simulink model "ADAS_Main"  (R2026a)
settings: Solver=FixedStepDiscrete  StopTime=5
InitFcn:
  | createLidarActorProfiles;
model workspace (MAT data in the model file):
  firstWarning = 1
  originalScenarioChecksum = '71EAF3DF157DF5A35F75811B676F8B0F'
undefined symbols (not defined in the file): driving, matlabshared
libraries: drivingscenarioandsensors x3, lidarlib x1
(part 4 of 6)

== matlab function ADAS_Main/Tracking_Prediction/Track_Lifecycle ==
  data: iState input; oState output; iCov input; iID input; iStatus input; iNextID input; iHits input; iTsu input; iR1 input; prevWin input uint32 size=512 1; prevAge input uint32 size=512 1; prevLost input double size=512 10; oCov output; oID output; oStatus output; oNextID output; oHits output; oTsu output; oR1 output; oWin output; oAge output; oLost output; lifeDiag output; iAttr input double size=512 3; oAttr output; oTrackAttributes output
function [oState, oCov, oID, oStatus, oNextID, oHits, oTsu, oR1, ...
          oWin, oAge, oLost, lifeDiag, oAttr, oTrackAttributes] = ...
    Track_Lifecycle(iState, iCov, iID, iStatus, iNextID, iHits, iTsu, iR1, ...
                    prevWin, prevAge, prevLost, iAttr)
%#codegen
% TRACK_LIFECYCLE  Stage 5: track lifecycle ONLY.
%   FREE -> TENTATIVE -> CONFIRMED -> COASTED -> LOST -> deleted (slot to FREE)
%
% THIS BLOCK DOES NOT: observe velocity, estimate acceleration, keep history,
% emit prediction horizons, rank threats, or make any manoeuvre decision.
% It does not touch the state estimate: it only changes STATUS and bookkeeping,
% and moves records between the active and lost tables.
%
% VELOCITY OBSERVATION REMAINS UNTOUCHED AND UNDECIDED. Velocity is never
% zeroed, never re-estimated and never used as a lifecycle criterion here.
%
% PLACEMENT: runs AFTER Track_Update, so Track_Update stays byte-identical
% (Stage-4 corrections are frozen). Its output feeds the Unit Delays.
%
% "MATCHED THIS FRAME" is detected as iTsu == 0. Track_Update sets tsu to 0 on a
% successful update and to prevTsu+dt otherwise, and a newly born track also has
% tsu 0 - which is correct, since birth is its first hit.
%
% CONFIRMATION - 2 of 3, NOT 2 consecutive
%   oWin is a 3-bit shift register, bit0 = most recent frame, 1 = hit.
%       win = bitand(bitshift(prevWin,1) + matched, 7)
%   CONFIRM  when popcount(win) >= 2
%   DELETE   when (age >= 2 and the last two frames are both misses)
%            or  (age >= 3 and popcount(win) < 2)   <- window closed, <2 hits
%   Confirmation is tested BEFORE deletion. Verified against all six frozen
%   sequences: hit-hit, hit-miss-hit, miss-hit-hit confirm; hit-miss-miss,
%   miss-hit-miss, miss-miss-* delete.
%
% COASTING
%   CONFIRMED + miss -> COASTED. A coasted track keeps its predicted state,
%   its velocity, and its covariance exactly as Track Prediction left them;
%   nothing is zeroed or reset. It keeps competing for association and stays
%   reported. COASTED + match -> CONFIRMED with the SAME TrackID.
%
% COASTED -> LOST (frozen criterion, no threat input)
%   sigma_assoc = sqrt(max(P11,P22)) of the current (predicted) covariance.
%   LOST when  KGATE * sigma_assoc >= WLANE  (3.03 * sigma >= 3.5 m).
%   The record is MOVED to the lost table and the active slot returns to FREE,
%   so a LOST record cannot participate in association - Track_Association
%   iterates the active table only and therefore needed no change.
%
% LOST retention (frozen, literal)
%   delete when TimeSinceUpdate >= T_LOST = 1.5 s.
%   NOTE: TimeSinceUpdate accumulates from the track's LAST UPDATE, not from
%   the moment it became LOST, so this gives 1.5 s of total post-update
%   retention rather than 1.5 s in addition to the coasting phase. This is the
%   literal frozen rule; the measured consequence is reported at the checkpoint.
%
% REACQUISITION - two different things
%   1. COASTED gets a match  -> CONFIRMED, SAME TrackID. Counted in NumReacquired.
%   2. A LOST object physically reappears -> must become a NEW track with a NEW
%      TrackID. NOT IMPLEMENTABLE HERE: recognising that a detection corresponds
%      to a lost record requires comparing it against the lost table, which is
%      association with LOST records and is explicitly forbidden. No flag is
%      fabricated. Reported as an open item.
%
% TrackID is uint32, monotonic, never reused, independent of slot index. A
% deleted or lost record never returns its ID to circulation.
%
% NO EVICTION anywhere: neither the active table nor the lost table ever removes
% an existing record to make room. Overflow is reported instead.
%
% SCENARIO INDEPENDENCE: consumes only track state, covariance and timing. No
% actor identity, class, count, trajectory, map or scenario geometry.

MAX_T  = 512;
MAX_L  = 512;          % MAX_TRACKS_LOST
NCOL_L = 10;
DT     = 0.1;
KGATE  = 3.03;
WLANE  = 3.5;
T_LOST = 1.5;
V_CONV = 0.875;

ST_FREE = uint8(0); ST_TENT = uint8(1); ST_CONF = uint8(2); ST_COAST = uint8(3);

oState  = zeros(MAX_T,4);
oCov    = zeros(MAX_T,10);
oID     = zeros(MAX_T,1,'uint32');
oStatus = zeros(MAX_T,1,'uint8');
oHits   = zeros(MAX_T,1,'uint32');
oTsu    = zeros(MAX_T,1);
oR1     = zeros(MAX_T,3);
% ---- additive: persistent LiDAR extent attributes, and the ICE-facing output --
% oAttr           [512x3]  state fed back through the Unit Delay
% oTrackAttributes[512x4]  Valid | Length | Width | TrustFlags
% A freed slot falls through the ~keep continue below, so BOTH arrays stay
% exactly zero for it. No extent is invented and no default size substituted.
oAttr            = zeros(MAX_T,3);
oTrackAttributes = zeros(MAX_T,4);
oWin    = zeros(MAX_T,1,'uint32');
oAge    = zeros(MAX_T,1,'uint32');
oLost   = zeros(MAX_L,NCOL_L);
oNextID = iNextID;
lifeDiag = zeros(1,12);

% ---- 1. age the lost table and retire expired records --------------------
nLostDel = 0;
for k = 1:MAX_L
    if prevLost(k,1) == 0
        continue                            % free lost slot
    end
    tsuL = prevLost(k,9) + DT;
    if tsuL >= T_LOST
        nLostDel = nLostDel + 1;            % retired; TrackID never returns
        continue
    end
    for c = 1:NCOL_L
        oLost(k,c) = prevLost(k,c);
    end
    oLost(k,9) = tsuL;
end

% ---- 2. lifecycle transitions on the active table ------------------------
nTent = 0; nConf = 0; nCoast = 0; nDelT = 0; nConfTr = 0; nReacq = 0;
nToLost = 0; lostOvf = 0; nLostDrop = 0; nConv = 0; nExpOnEntry = 0;

for t = 1:MAX_T
    st = iStatus(t);
    if st == ST_FREE
        continue                            % slot stays entirely zero
    end

    matched = 0;
    if iTsu(t) == 0
        matched = 1;
    end
    w  = bitand(bitshift(uint32(prevWin(t)),1) + uint32(matched), uint32(7));
    ag = prevAge(t) + uint32(1);
    pc = bitand(w,uint32(1)) + bitand(bitshift(w,-1),uint32(1)) + bitand(bitshift(w,-2),uint32(1));

    keep = true;
    toLost = false;

    if st == ST_TENT
        if pc >= 2
            st = ST_CONF; nConfTr = nConfTr + 1;
        elseif (ag >= 2 && bitand(w,uint32(3)) == 0) || (ag >= 3 && pc < 2)
            keep = false; nDelT = nDelT + 1;
        end
    elseif st == ST_CONF
        if matched == 0
            st = ST_COAST;
        end
    else                                    % ST_COAST
        if matched == 1
            st = ST_CONF; nReacq = nReacq + 1;
        end
    end

    if keep && st == ST_COAST
        s1 = iCov(t,1); s2 = iCov(t,5);
        sm = s1; if s2 > sm, sm = s2; end
        if sm < 0, sm = 0; end
        if KGATE*sqrt(sm) >= WLANE
            toLost = true; keep = false;
        end
    end

    if toLost && iTsu(t) >= T_LOST
        % already past the retention limit at the moment of transfer - the
        % literal rule retires it immediately rather than holding it a frame
        nLostDel = nLostDel + 1;
        nExpOnEntry = nExpOnEntry + 1;
        toLost = false;
    end

    if toLost
        slot = 0;
        for k = 1:MAX_L
            if oLost(k,1) == 0, slot = k; break; end
        end
        if slot == 0
            lostOvf = 1; nLostDrop = nLostDrop + 1;   % NEVER evict an existing record
        else
            oLost(slot,1)  = double(iID(t));
            oLost(slot,2)  = iState(t,1);
            oLost(slot,3)  = iState(t,2);
            oLost(slot,4)  = iState(t,3);
            oLost(slot,5)  = iState(t,4);
            oLost(slot,6)  = iCov(t,1);
            oLost(slot,7)  = iCov(t,5);
            oLost(slot,8)  = iCov(t,2);
            oLost(slot,9)  = iTsu(t);
            oLost(slot,10) = double(ag);
            nToLost = nToLost + 1;
        end
    end

    if ~keep
        continue                            % slot returns to FREE (all zeros)
    end

    for c = 1:4,  oState(t,c) = iState(t,c); end
    for c = 1:10, oCov(t,c)   = iCov(t,c);   end
    for c = 1:3,  oR1(t,c)    = iR1(t,c);    end
    for c = 1:3,  oAttr(t,c)  = iAttr(t,c);  end
    oTrackAttributes(t,1) = 1;                  % Valid == post-lifecycle validity
    oTrackAttributes(t,2) = iAttr(t,1);         % Length
    oTrackAttributes(t,3) = iAttr(t,2);         % Width
    oTrackAttributes(t,4) = iAttr(t,3);         % TrustFlags, carried verbatim
    oID(t)     = iID(t);
    oStatus(t) = st;
    oHits(t)   = iHits(t);
    oTsu(t)    = iTsu(t);
    oWin(t)    = w;
    oAge(t)    = ag;

    if st == ST_TENT,  nTent  = nTent  + 1; end
    if st == ST_CONF,  nConf  = nConf  + 1; end
    if st == ST_COAST, nCoast = nCoast + 1; end
    if sqrt(iCov(t,8)) < V_CONV && sqrt(iCov(t,10)) < V_CONV
        nConv = nConv + 1;                  % derived, never a lifecycle criterion
    end
end

nLostNow = 0;
for k = 1:MAX_L
    if oLost(k,1) ~= 0, nLostNow = nLostNow + 1; end
end

lifeDiag(1)  = nTent;
lifeDiag(2)  = nConf;
lifeDiag(3)  = nCoast;
lifeDiag(4)  = nLostNow;
lifeDiag(5)  = nDelT + nLostDel;
lifeDiag(6)  = nDelT;
lifeDiag(7)  = nConfTr;
lifeDiag(8)  = nReacq;
lifeDiag(9)  = nToLost;
lifeDiag(10) = lostOvf;
lifeDiag(11) = nLostDrop;
lifeDiag(12) = nConv;

end

== matlab function ADAS_Main/Tracking_Prediction/Track_History ==
  data: trkState input; hist output; trkID input; trkStatus input; trkTsu input; simTime input; prevHist input double size=512 30 4; prevRing input uint32 size=512 1; ringIdx output; validCount output; histSpan output
function [hist, ringIdx, validCount, histSpan] = ...
    Track_History(trkState, trkID, trkStatus, trkTsu, simTime, prevHist, prevRing)
%#codegen
% TRACK_HISTORY  Stage 6: per-track temporal history ONLY.
%
% THIS BLOCK DOES NOT: estimate acceleration, emit prediction horizons, run
% Behavior/Intention, Risk, Planning or Controller, observe velocity, or do any
% LOST-track re-identification. It does not touch the state estimate, the
% lifecycle, or any Stage-3/4/5 contract - it only records where each active
% track has been.
%
% Tracking's own recursive estimator needs no history. This buffer exists to
% give Behavior/Intention temporal information downstream.
%
% LAYOUT (frozen)
%   hist [512 x 30 x 4] double   channel 1 = X
%                                channel 2 = Y
%                                channel 3 = Valid (1 measured, 0 predicted)
%                                channel 4 = timestamp (s, actual sim time)
%   30 samples at dt = 0.1 s  ->  3.0 s of coverage.
%   ringIdx [512 x 1] uint32     index of the MOST RECENT sample, 1..30; 0 = empty
%
% RING BEHAVIOUR
%   The ring advances EVERY frame for every active track, whether or not a
%   measurement arrived. The temporal grid therefore stays uniform:
%   t, t-dt, t-2dt, ... Valid samples are never compacted together, so a gap
%   remains visible as a run of Valid = 0 rather than being closed up.
%   On the 31st write the oldest sample is overwritten deterministically.
%
% VALID
%   Valid = 1 only when the track received a measurement this frame, detected as
%   trkTsu == 0 (Track_Update zeroes it on a successful update and on birth).
%   A COASTED track - or a TENTATIVE track that missed - still gets a sample
%   written with its PREDICTED X/Y, but marked Valid = 0. A prediction is never
%   recorded as a measurement.
%
% STATUS INDEPENDENCE
%   Storage does not depend on confirmation status. TENTATIVE, CONFIRMED and
%   COASTED tracks all keep history. History is never deleted for being
%   unconfirmed, and never ranked or filtered - every active slot has its own
%   independent buffer.
%
% FREE SLOTS AND SLOT REUSE
%   A slot whose status is FREE has its entire history zeroed and ringIdx set to
%   0. Because Track_Lifecycle frees a slot in the very output this block
%   consumes, the FREE state is always observed before any new track can occupy
%   that slot, so a new occupant always starts from a cleared buffer. Old and
%   new trajectories are therefore never spliced.
%
% LOST
%   A track entering LOST leaves the active table, so its slot reads FREE here
%   and its history is discarded. No history is kept for LOST records and none
%   is ever carried into a future track.
%
% TrackID vs SLOT
%   History follows the SLOT. trkID is carried only so downstream can label the
%   buffer; it is never assumed equal to the slot index.
%
% DERIVED METADATA (the only two exposed at this stage)
%   validCount [512 x 1]  number of Valid == 1 samples, 0..30. Coasted and
%                         empty samples are NOT counted.
%   histSpan   [512 x 1]  newest valid timestamp minus oldest valid timestamp,
%                         computed from the STORED TIMESTAMPS, not from the
%                         valid-sample count. Fewer than two valid samples -> 0.
%                         So valid,valid,invalid,invalid,valid spans 0.4 s, not
%                         the 0.2 s a count-based formula would give.
%
% SCENARIO INDEPENDENCE: consumes only track state, status, timing and the
% simulation clock. No actor identity, class, count, map or scenario geometry.

MAX_T = 512;
NS    = 30;

hist       = zeros(MAX_T, NS, 4);
ringIdx    = zeros(MAX_T, 1, 'uint32');
validCount = zeros(MAX_T, 1);
histSpan   = zeros(MAX_T, 1);

ts = simTime;
if ~isfinite(ts), ts = 0; end

for t = 1:MAX_T
    if trkStatus(t) == 0
        continue                    % FREE: history and ring stay exactly zero
    end

    % ---- advance the ring every frame, measured or not
    ri = double(prevRing(t)) + 1;
    if ri > NS, ri = 1; end
    if ri < 1,  ri = 1; end

    for s = 1:NS
        for c = 1:4
            hist(t,s,c) = prevHist(t,s,c);
        end
    end

    vflag = 0;
    if trkTsu(t) == 0
        vflag = 1;                  % measured this frame
    end
    hist(t,ri,1) = trkState(t,1);
    hist(t,ri,2) = trkState(t,2);
    hist(t,ri,3) = vflag;
    hist(t,ri,4) = ts;
    ringIdx(t)   = uint32(ri);

    % ---- derived metadata, from the stored timestamps
    nv = 0; tmin = 0; tmax = 0; first = true;
    for s = 1:NS
        if hist(t,s,3) == 1
            nv = nv + 1;
            tv = hist(t,s,4);
            if first
                tmin = tv; tmax = tv; first = false;
            else
                if tv < tmin, tmin = tv; end
                if tv > tmax, tmax = tv; end
            end
        end
    end
    validCount(t) = nv;
    if nv >= 2
        histSpan(t) = tmax - tmin;
    else
        histSpan(t) = 0;
    end
end

end

== matlab function ADAS_Main/Tracking_Prediction/Prediction_Horizons ==
  data: trkState input; trkPred output; trkCov input; trkStatus input
function trkPred = Prediction_Horizons(trkState, trkCov, trkStatus)
%#codegen
% PREDICTION_HORIZONS  Stage 7: pure kinematic projection of each active track
% onto a fixed ladder of future times. NOTHING ELSE.
%
% THIS BLOCK DOES NOT: estimate acceleration, fit anything to Track History,
% classify manoeuvres, produce lane-change / braking / cut-in / overtaking
% likelihoods, compute TTC, collision probability, risk or threat, or propose
% ego trajectories. Those belong to Behavior/Intention, the Risk Engine and
% Planning respectively. It answers only "where could this object be under the
% existing CV model", never "what will it choose to do".
%
% It is a PURE FUNCTION of the current track state - stateless, no Unit Delay.
% It does not modify Track_History, Track_Lifecycle, Track_Update or any
% Stage-3..6 contract, and velocity observation is untouched.
%
% EGO FRAME
%   The input state is already expressed in the current ego-compensated frame.
%   No further ego compensation is applied, no future ego motion is assumed, and
%   no ego manoeuvre is presumed. Outputs are target states relative to the
%   CURRENT compensated tracking frame.
%
% MEAN
%   x_h = F(h)*x ,  F(h) = [1 0 h 0; 0 1 0 h; 0 0 1 0; 0 0 0 1]
%
% COVARIANCE - OPTION B (approved): exact closed-form evaluation of the
% ALREADY FROZEN discrete-time model. This is NOT a new covariance model; it is
% the algebraic value of
%       P_N = F^N P (F^N)' + sum_{j=0}^{N-1} F^j Q(dt) (F^j)'
% computed without numerically iterating. With a = dt^4/4, b = dt^3/2, c = dt^2
% and N = h/dt (exactly integral for all seven horizons: 5 10 15 20 30 40 50):
%       Q11 = q*[ N*a + b*dt*N*(N-1) + c*dt^2*(N-1)*N*(2*N-1)/6 ]
%       Q12 = q*[ N*b + c*dt*N*(N-1)/2 ]
%       Q22 = q*[ N*c ]
%   Verified against explicit repeated Q(dt) propagation on all 16 elements and
%   all seven horizons: max |dQ| 2.13e-14, max |dP| 7.11e-15, and over 500
%   random PD covariances max |dP| 4.55e-13.
%
%   The single-step form q*h^4/4 is DELIBERATELY NOT USED - it does not match the
%   frozen Stage-2 discrete process model and would inflate sigma at 5 s from
%   6.48 m to 37.56 m.
%
% OUTPUT  trkPred [512 x 7 x 7] double, indexed (track, horizon, field)
%   horizon index 1..7 -> 0.5 1.0 1.5 2.0 3.0 4.0 5.0 s
%   field   index 1..7 -> 1 X, 2 Y, 3 Vx, 4 Vy, 5 PosCovXX, 6 PosCovYY, 7 PosCovXY
%   Both trailing dimensions are 7; the ordering above is the contract.
%
% COVERAGE
%   Every ACTIVE track is predicted - TENTATIVE, CONFIRMED and COASTED alike.
%   No ranking, no filtering, no "primary target", no nearest/front/highest-score
%   selection. If 107 tracks are active, all 107 get the full ladder. LOST tracks
%   are not in the active table and so receive nothing. FREE rows stay zero.
%
% UNCERTAINTY
%   Covariance grows naturally with the horizon and is never clamped, shrunk or
%   cosmetically adjusted, and a large covariance is never a reason to drop a
%   track - lifecycle already made that call. A track with
%   VelocityConverged = false keeps its large velocity covariance, which
%   propagates into the position covariance exactly as the model dictates; its
%   Vx = Vy = 0 placeholder is NOT treated as stationary and its future velocity
%   is NOT zeroed. Downstream interprets the uncertainty.
%
% SCENARIO INDEPENDENCE: consumes only track state, covariance and status. No
% actor identity, class, count, map or scenario geometry.

MAX_T = 512;
NH    = 7;
NFLD  = 7;
DT    = 0.1;
QA    = 9.0;                 % m^2/s^4, frozen
P_FLOOR_POS = 1e-6;          % existing floor, applied only if violated

trkPred = zeros(MAX_T, NH, NFLD);

hor = [0.5 1.0 1.5 2.0 3.0 4.0 5.0];
aa = DT^4/4;  bb = DT^3/2;  cc = DT^2;

for k = 1:NH
    h = hor(k);
    N = h/DT;
    Nr = floor(N + 0.5);
    if Nr < 1, Nr = 1; end
    Nd = double(Nr);

    q11 = QA*( Nd*aa + bb*DT*Nd*(Nd-1) + cc*DT*DT*(Nd-1)*Nd*(2*Nd-1)/6 );
    q12 = QA*( Nd*bb + cc*DT*Nd*(Nd-1)/2 );   %#ok<NASGU> same-axis pos/vel term,
    % retained for documentation of the full Q_acc; the position block only
    % needs Q_acc(1,1)=q11 and Q_acc(2,2)=q11, and Q_acc(1,2)=0.
    q22 = QA*( Nd*cc );

    for t = 1:MAX_T
        if trkStatus(t) == 0
            continue                     % FREE row stays zero
        end

        x1 = trkState(t,1); x2 = trkState(t,2);
        x3 = trkState(t,3); x4 = trkState(t,4);

        p11 = trkCov(t,1); p12 = trkCov(t,2); p13 = trkCov(t,3); p14 = trkCov(t,4);
        p22 = trkCov(t,5); p23 = trkCov(t,6); p24 = trkCov(t,7);
        p33 = trkCov(t,8); p34 = trkCov(t,9); p44 = trkCov(t,10);

        % ---- mean: x_h = F(h)*x
        m1 = x1 + h*x3;
        m2 = x2 + h*x4;
        m3 = x3;
        m4 = x4;

        % ---- position block of F(h)*P*F(h)' , then + Q_acc
        c11 = p11 + 2*h*p13 + h*h*p33 + q11;
        c22 = p22 + 2*h*p24 + h*h*p44 + q11;
        % NOTE: Q_acc(1,2) is ZERO - q12 is the position/velocity cross term of
        % the SAME axis (Q_acc(1,3)), not the x-y position cross term. It must
        % NOT be added here.
        c12 = p12 + h*p14 + h*p23 + h*h*p34;

        if ~isfinite(c11) || c11 < P_FLOOR_POS, c11 = P_FLOOR_POS; end
        if ~isfinite(c22) || c22 < P_FLOOR_POS, c22 = P_FLOOR_POS; end
        if ~isfinite(c12), c12 = 0; end
        if ~isfinite(m1), m1 = 0; end
        if ~isfinite(m2), m2 = 0; end
        if ~isfinite(m3), m3 = 0; end
        if ~isfinite(m4), m4 = 0; end

        trkPred(t,k,1) = m1;
        trkPred(t,k,2) = m2;
        trkPred(t,k,3) = m3;
        trkPred(t,k,4) = m4;
        trkPred(t,k,5) = c11;
        trkPred(t,k,6) = c22;
        trkPred(t,k,7) = c12;
    end
end

end

== matlab function ADAS_Main/Behavior_ICE/ICE_Evaluate ==
  data: TrackState input; Verdict3 output; TrackCov input; TrackID input; TrackStatus input; TrackAttributes input; EgoKinematics input; M_adm output; N_adm output; N_inadm output; InadmIDs output; InadmReason output; InadmOverflow output; AdmVacuous output; Bind output; N_active output; N_clear output; M_res output; ResVacuous output
function [Verdict3, M_adm, N_adm, N_inadm, InadmIDs, InadmReason, ...
          InadmOverflow, AdmVacuous, Bind, N_active, N_clear, M_res, ResVacuous] = ...
    ICE_Evaluate(TrackState, TrackCov, TrackID, TrackStatus, TrackAttributes, EgoKinematics) %#codegen
%ICE_EVALUATE  Fixed-size ICE, Simulink MATLAB Function compatible.
%
%   Functionally equivalent to ice_adm(ice_core(...)). The reference pair
%   ice_core.m / ice_adm.m / ice_par.m remains the ORACLE; this file must
%   reproduce them. No mathematics, parameter, semantic or threshold changed.
%
%   FIXED SIZE ONLY. No find(), no unique(), no sort(), no varsize, no heap.
%   See ICE_FIXEDSIZE_NOTES in the design document for the three replacements.
%
%   Ego model, per approved decisions:
%     egoV   = EgoKinematics(1)   planar ego speed        (D3)
%     egoPsi = 0                  pinned interface invariant (D5)
%     straight nominal candidate lattice                   (D4)
%     EgoKinematics(2) (yaw rate) carried but NOT consumed (D5/approved item 5)

%% ---- constants, copied VERBATIM from ice_par.m -------------------------
NT   = 512;                                   % PAR.capN
HS   = [0.5 1.0 1.5 2.0 3.0 4.0 5.0];         % PAR.hs
H    = 7;
O    = 4;                                     % PAR.O
NANG = 8;                                     % PAR.nAng
NRAD = 4;                                     % PAR.nRad
MC   = NANG*NRAD;                             % 32 candidates per sector
CLEVEL = 9.21;
U      = 8.0;
VMAX   = 40.0;
U_EGO  = 8.0;
R_EGO  = 3.9906;
ASPECT = 10.0;
OCCL   = 2.0;
UNTRUST= 2.0;
THINFL = 0.6;
ACTTOL = 1e-9;
BC     = 8;                                   % PAR.bindCap
IC     = 32;                                  % InadmIDs capacity (approved)
NOAGENT= inf;                                 % PAR.noAgentMargin
FL_THIN      = 4;
FL_UNTRUSTED = 8;

EGOV   = EgoKinematics(1);                    % D3
% egoPsi is pinned to 0 (D5). The rotation R(-0) is the exact identity, so
% it is omitted rather than multiplied; equivalence is asserted by test.

%% ---- outputs preallocated (fixed size) ---------------------------------
Verdict3      = zeros(O,H,'int8');
M_adm         = zeros(O,H);
N_active      = zeros(O,H,'uint16');
N_clear       = zeros(O,H,'uint16');
M_res         = zeros(O,H);
ResVacuous    = false(O,H);
Bind          = zeros(O,H,BC,'uint32');
InadmIDs      = zeros(IC,1,'uint32');
InadmReason   = zeros(IC,1,'uint8');
InadmOverflow = false;

%% ---- stage 1: admissibility over ALL 512 slots -------------------------
% Reason bits: 1 EXTENT | 2 COVARIANCE | 4 OTHER
live   = false(NT,1);
reason = zeros(NT,1,'uint8');
for t = 1:NT
    if TrackStatus(t) == 0
        continue
    end
    live(t) = true;
    r = uint8(0);

    if TrackAttributes(t,1) ~= 1
        r = bitor(r, uint8(4));
    end

    L = TrackAttributes(t,2);
    W = TrackAttributes(t,3);
    if ~isfinite(L) || ~isfinite(W) || L <= 0 || W <= 0
        r = bitor(r, uint8(1));
    end

    p11 = TrackCov(t,1); p12 = TrackCov(t,2);
    q11 = TrackCov(t,3); q12 = TrackCov(t,4);
    p22 = TrackCov(t,5);
    q21 = TrackCov(t,6); q22 = TrackCov(t,7);
    v11 = TrackCov(t,8); v12 = TrackCov(t,9); v22 = TrackCov(t,10);
    finite10 = isfinite(p11) && isfinite(p12) && isfinite(q11) && isfinite(q12) && ...
               isfinite(p22) && isfinite(q21) && isfinite(q22) && ...
               isfinite(v11) && isfinite(v12) && isfinite(v22);
    if ~finite10 || ~isPD2f(p11,p12,p12,p22)
        r = bitor(r, uint8(2));
    else
        for k = 1:H
            h = HS(k);
            s11 = p11 + 2*h*q11 + h*h*v11;
            s12 = p12 + h*(q12 + q21) + h*h*v12;
            s22 = p22 + 2*h*q22 + h*h*v22;
            if ~isPD2f(s11,s12,s12,s22)
                r = bitor(r, uint8(2));
                break
            end
        end
    end
    reason(t) = r;
end

adm = live & (reason == 0);
nAdm = 0; nInadm = 0; nFill = 0;
for t = 1:NT
    if ~live(t), continue; end
    if reason(t) == 0
        nAdm = nAdm + 1;
    else
        nInadm = nInadm + 1;
        if nFill < IC                      % slot order; NO ranking
            nFill = nFill + 1;
            InadmIDs(nFill)    = TrackID(t);
            InadmReason(nFill) = reason(t);
        else
            InadmOverflow = true;
        end
    end
end
N_adm      = uint16(nAdm);
N_inadm    = uint16(nInadm);
AdmVacuous = (nAdm == 0);

%% ---- stage 2: per-agent envelopes, all 512 slots -----------------------
rFoot    = zeros(NT,1);
cAx = zeros(NT,H); cAy = zeros(NT,H); rA = zeros(NT,H);
cBx = zeros(NT,H); cBy = zeros(NT,H); rB = zeros(NT,H);
resolved = false(NT,H);

for t = 1:NT
    if ~adm(t), continue; end

    L = TrackAttributes(t,2);
    W = TrackAttributes(t,3);
    fl = uint32(max(TrackAttributes(t,4),0));
    base = 0.5*sqrt(L*L + W*W);
    if bitand(fl, uint32(FL_UNTRUSTED)) > 0
        base = base * UNTRUST;
    end
    if bitand(fl, uint32(FL_THIN)) > 0
        base = max(base, THINFL);
    end
    cap = ASPECT * 0.5 * min(L,W);
    rFoot(t) = min(base + OCCL, max(base, cap));

    p11 = TrackCov(t,1); p12 = TrackCov(t,2);
    q11 = TrackCov(t,3); q12 = TrackCov(t,4);
    p22 = TrackCov(t,5);
    q21 = TrackCov(t,6); q22 = TrackCov(t,7);
    v11 = TrackCov(t,8); v12 = TrackCov(t,9); v22 = TrackCov(t,10);

    r0 = sqrt(CLEVEL * lmax2f(p11,p12,p12,p22));
    for k = 1:H
        h = HS(k);
        s11 = p11 + 2*h*q11 + h*h*v11;
        s12 = p12 + h*(q12 + q21) + h*h*v12;
        s22 = p22 + 2*h*q22 + h*h*v22;
        rEpi = sqrt(CLEVEL * lmax2f(s11,s12,s12,s22));
        cAx(t,k) = TrackState(t,1) + h*TrackState(t,3);
        cAy(t,k) = TrackState(t,2) + h*TrackState(t,4);
        rA(t,k)  = rEpi + 0.5*U*h*h + rFoot(t);
        cBx(t,k) = TrackState(t,1);
        cBy(t,k) = TrackState(t,2);
        rB(t,k)  = r0 + VMAX*h + rFoot(t);
        resolved(t,k) = (rEpi < 0.5*min(L,W));
    end
end

%% ---- stage 3: candidates and max-min -----------------------------------
dA  = zeros(MC,NT);
dB  = zeros(MC,NT);
Dm  = zeros(MC,NT);
Dr  = zeros(MC,NT);
d1  = zeros(MC,1);
i1  = zeros(MC,1);
d2  = zeros(MC,1);
activeFlag = false(NT,1);
bidbuf = zeros(BC,1,'uint32');

for k = 1:H
    h      = HS(k);
    egoNom = EGOV*h;                        % D3/D4: straight nominal
    Rreach = 0.5*U_EGO*h*h;
    for o = 1:O
        w  = 2*pi/O;
        a0 = -pi + (o-1)*w;

        % ---- REPLACEMENT 1 for find(): mask, never gather -------------
        % every non-admissible column is +Inf so it can never attain a min
        for m = 1:MC
            ia = floor((m-1)/NRAD) + 1;     % meshgrid(ang,rad) column-major
            ir = m - (ia-1)*NRAD;
            ang = a0 + (ia - 0.5)*(w/NANG);
            rad = (ir/NRAD)*Rreach;
            cx  = egoNom + rad*cos(ang);
            cy  =          rad*sin(ang);
            for t = 1:NT
                if ~adm(t)
                    dA(m,t) = inf; dB(m,t) = inf; Dm(m,t) = inf; Dr(m,t) = inf;
                    continue
                end
                ax = cx - cAx(t,k); ay = cy - cAy(t,k);
                bx = cx - cBx(t,k); by = cy - cBy(t,k);
                da = hypot(ax,ay) - R_EGO - rA(t,k);
                db = hypot(bx,by) - R_EGO - rB(t,k);
                dA(m,t) = da; dB(m,t) = db;
                dm = da; if db > dm, dm = db; end
                Dm(m,t) = dm;
                if resolved(t,k), Dr(m,t) = dm; else, Dr(m,t) = inf; end
            end
        end

        % row minima and second minima
        Mv = -inf; nClear = 0;
        for m = 1:MC
            bv = inf; bi = 0;
            for t = 1:NT
                if Dm(m,t) < bv, bv = Dm(m,t); bi = t; end
            end
            d1(m) = bv; i1(m) = bi;
            sv = inf;
            for t = 1:NT
                if t == bi, continue; end
                if Dm(m,t) < sv, sv = Dm(m,t); end
            end
            d2(m) = sv;
            if bv > Mv, Mv = bv; end
            if bv > 0,  nClear = nClear + 1; end
        end

        % ---- REPLACEMENT 2 for unique(): set membership by flag -------
        for t = 1:NT, activeFlag(t) = false; end
        for m = 1:MC
            if d2(m) > Mv + ACTTOL && i1(m) > 0
                activeFlag(i1(m)) = true;
            end
        end

        % ---- REPLACEMENT 3 for sort(): bounded ascending insertion ----
        % keeps the BC smallest TrackIDs in ascending order, exactly as
        % sort(...) followed by truncation to BC does in the reference
        nb = 0; nActive = 0;
        for b = 1:BC, bidbuf(b) = uint32(0); end
        for t = 1:NT
            if ~activeFlag(t), continue; end
            nActive = nActive + 1;
            v = TrackID(t);
            pos = nb + 1;
            for b = 1:BC
                if b <= nb && v < bidbuf(b)
                    pos = b; break
                end
            end
            if pos <= BC
                last = nb; if last > BC-1, last = BC-1; end
                for b = last:-1:pos
                    bidbuf(b+1) = bidbuf(b);
                end
                bidbuf(pos) = v;
                if nb < BC, nb = nb + 1; end
            end
        end

        % resolved-agent bracket
        Mr = -inf; anyRes = false;
        for m = 1:MC
            rv = inf;
            for t = 1:NT
                if Dr(m,t) < rv, rv = Dr(m,t); end
            end
            if rv > Mr, Mr = rv; end
        end
        for t = 1:NT
            if adm(t) && resolved(t,k), anyRes = true; break; end
        end

        % ---- outputs -------------------------------------------------
        if nAdm == 0
            M_adm(o,k)      = NOAGENT;
            N_clear(o,k)    = uint16(MC);
            N_active(o,k)   = uint16(0);
        else
            M_adm(o,k)      = Mv;
            N_clear(o,k)    = uint16(nClear);
            N_active(o,k)   = uint16(nActive);
        end
        if anyRes
            M_res(o,k)      = Mr;
            ResVacuous(o,k) = false;
        else
            M_res(o,k)      = NOAGENT;
            ResVacuous(o,k) = true;
        end
        for b = 1:BC
            Bind(o,k,b) = bidbuf(b);
        end

        % three-state certification (approved semantics)
        if M_adm(o,k) <= 0
            Verdict3(o,k) = int8(2);                    % BLOCKED
        elseif nInadm == 0
            Verdict3(o,k) = int8(1);                    % AVAILABLE
        else
            Verdict3(o,k) = int8(0);                    % UNKNOWN
        end
    end
end
end

%% ================= local helpers =================
function tf = isPD2f(a,b,c,d)
tf = isfinite(a) && isfinite(d) && isfinite(b) && ...
     a > 0 && d > 0 && (a*d - b*c) > 0;
end

function l = lmax2f(a,b,c,d)
tr = a + d;
dt = a*d - b*c;
l  = (tr + sqrt(max(tr*tr - 4*dt, 0)))/2;
end

== matlab function ADAS_Main/Behavior_Risk/Risk_Evaluate ==
  data: Bind input; EffLimiterCount output; M_adm input; AdmVacuous input; PrevM input double size=[4 7]; PrevIDs input uint32 size=[224 1]; PrevN input uint16 size=[1 1]; FirstFrame input boolean size=[1 1]; TopLimiterShare output; TopLimiterID output; MarginTrend output; LimiterEnter output; LimiterExit output; RiskValid output; PrevM_out output; PrevIDs_out output; PrevN_out output
function [EffLimiterCount, TopLimiterShare, TopLimiterID, MarginTrend, ...
          LimiterEnter, LimiterExit, RiskValid, PrevM_out, PrevIDs_out, PrevN_out] = ...
          Risk_Evaluate(Bind, M_adm, AdmVacuous, PrevM, PrevIDs, PrevN, FirstFrame) %#codegen
%RISK_EVALUATE  Fixed-size Constraint Structure Estimation.
%
%   Functionally identical to risk_core.m, which remains the oracle. Written
%   for a Simulink MATLAB Function block: every array is fixed size, every
%   loop is statically bounded, and no forbidden construct appears.
%
%   NOT USED: find, unique, sort, cell, persistent, dynamic growth,
%   variable-size arrays, dynamic containers.
%
%   Bounded-cost structure (worst case, all 224 Bind entries distinct):
%     per-sector histogram   4 x 56 x 56           =  12,544 comparisons
%     scene-wide set build   224 x 224 scan+shift  ~ 100,352
%     enter / exit           2 x 224 x 224         = 100,352
%   All statically bounded; no data-dependent allocation anywhere.

%% ---- fixed dimensions -------------------------------------------------
O   = 4;
H   = 7;
J   = 8;
CAP = 224;                                  % O*H*J - Bind can hold no more

%% ---- outputs preallocated at fixed size -------------------------------
EffLimiterCount = zeros(O,1);
TopLimiterShare = zeros(O,1);
TopLimiterID    = zeros(O,1,'uint32');
MarginTrend     = zeros(O,H);
LimiterEnter    = uint16(0);
LimiterExit     = uint16(0);
PrevIDs_out     = zeros(CAP,1,'uint32');

pn = double(PrevN);
if pn < 0,   pn = 0;   end
if pn > CAP, pn = CAP; end

%% ---- scene-wide distinct active set A_t -------------------------------
% Built in ASCENDING TrackID order by bounded insertion, so that
% PrevIDs_out matches risk_core's unique() output element for element.
At = zeros(CAP,1,'uint32');
nA = 0;
for o = 1:O
    for k = 1:H
        for j = 1:J
            v = Bind(o,k,j);
            if v == 0
                continue
            end
            found = false;
            pos   = nA + 1;
            for a = 1:CAP
                if a > nA
                    break
                end
                if At(a) == v
                    found = true;
                    break
                elseif At(a) > v
                    pos = a;
                    break
                end
            end
            if ~found && nA < CAP
                for b = CAP-1:-1:1                 % bounded shift
                    if b >= pos && b <= nA
                        At(b+1) = At(b);
                    end
                end
                At(pos) = v;
                nA = nA + 1;
            end
        end
    end
end

%% ---- state update (always, so the next valid frame has history) -------
PrevM_out = M_adm;
for a = 1:CAP
    if a <= nA
        PrevIDs_out(a) = At(a);
    end
end
PrevN_out = uint16(nA);

%% ---- validity ---------------------------------------------------------
% Matches risk_core, including the cross-frame finiteness guard: a frame
% following an AdmVacuous frame carries +Inf in PrevM and would otherwise
% produce -Inf in MarginTrend.
histFinite = true;
curFinite  = true;
for o = 1:O
    for k = 1:H
        if ~isfinite(PrevM(o,k)), histFinite = false; end
        if ~isfinite(M_adm(o,k)), curFinite  = false; end
    end
end
RiskValid = (~FirstFrame) && (~AdmVacuous) && histFinite && curFinite;

if ~RiskValid
    return                                   % outputs already zero
end

%% ---- 1. sector attribution -------------------------------------------
for o = 1:O
    tids = zeros(CAP,1,'uint32');            % fixed histogram table
    tcnt = zeros(CAP,1);
    nE   = 0;
    tot  = 0;

    for k = 1:H
        for j = 1:J
            v = Bind(o,k,j);
            if v == 0
                continue
            end
            tot = tot + 1;
            hit = 0;
            for a = 1:CAP
                if a > nE
                    break
                end
                if tids(a) == v
                    hit = a;
                    break
                end
            end
            if hit > 0
                tcnt(hit) = tcnt(hit) + 1;
            elseif nE < CAP
                nE = nE + 1;
                tids(nE) = v;
                tcnt(nE) = 1;
            end
        end
    end

    if tot == 0
        continue                             % empty sector: 0 sentinel
    end

    % sum of squared integer counts - exact, and order-independent, so the
    % encounter order here matches risk_core's ascending order bit for bit
    sumsq  = 0;
    bestN  = -1;
    bestID = uint32(0);
    for a = 1:CAP
        if a > nE
            break
        end
        c = tcnt(a);
        sumsq = sumsq + c*c;
        % strictly greater count wins; equal count resolves to the SMALLEST
        % TrackID, matching risk_core's first-maximum over ascending ids
        if (c > bestN) || (c == bestN && tids(a) < bestID)
            bestN  = c;
            bestID = tids(a);
        end
    end

    EffLimiterCount(o) = (tot*tot) / sumsq;
    TopLimiterShare(o) = bestN / tot;
    TopLimiterID(o)    = bestID;
end

%% ---- 2. margin trend --------------------------------------------------
for o = 1:O
    for k = 1:H
        MarginTrend(o,k) = M_adm(o,k) - PrevM(o,k);
    end
end

%% ---- 3. limiter set transition ---------------------------------------
en = 0;
for a = 1:CAP
    if a > nA
        break
    end
    hit = false;
    for b = 1:CAP
        if b > pn
            break
        end
        if PrevIDs(b) == At(a)
            hit = true;
            break
        end
    end
    if ~hit
        en = en + 1;
    end
end

ex = 0;
for b = 1:CAP
    if b > pn
        break
    end
    hit = false;
    for a = 1:CAP
        if a > nA
            break
        end
        if At(a) == PrevIDs(b)
            hit = true;
            break
        end
    end
    if ~hit
        ex = ex + 1;
    end
end

LimiterEnter = uint16(en);
LimiterExit  = uint16(ex);
end

== matlab function ADAS_Main/Behavior_Planning/Plan_Generate ==
  data: Verdict3 input; TrajX output; M_adm input; N_inadm input; AdmVacuous input; TrackState input; TrackCov input; TrackStatus input; TrackAttributes input; TrackID input; EgoKinematics input; MarginTrend input; EffLimiterCount input; RiskValid input; TrajY output; TrajV output; TrajCurv output; TrajValid output; ManoeuvreLabel output; FallbackActive output; NumFeasible output; NumClear output; NumTracksEvaluated output; RejectIDs output; PlanStale output; CandX output; CandY output; CandV output; CandCurv output; CandValid output
function [TrajX, TrajY, TrajV, TrajCurv, TrajValid, ManoeuvreLabel, ...
          FallbackActive, NumFeasible, NumClear, NumTracksEvaluated, ...
          RejectIDs, PlanStale, ...
          CandX, CandY, CandV, CandCurv, CandValid] = Plan_Generate( ...
          Verdict3, M_adm, N_inadm, AdmVacuous, TrackState, TrackCov, ...
          TrackStatus, TrackAttributes, TrackID, EgoKinematics, ...
          MarginTrend, EffLimiterCount, RiskValid) %#codegen
%PLAN_GENERATE  Planning Stage 1 - CANDIDATE GENERATION ONLY.
%
%   Generates the fixed 35 x 11 candidate trajectory set from the current ego
%   speed. NOTHING is selected, evaluated, filtered or checked for feasibility.
%
%   NOT IMPLEMENTED (each has its own approved later stage):
%     Plan_Feasibility, Plan_Envelopes, Plan_Evaluate, Plan_Select, fallback,
%     Planning state, Risk logic, lane/drivable-space reasoning.
%
%   The candidate set is exposed to Stage 2. The 12 PUBLIC outputs remain in
%   their Stage-0 safe stub state: TrajValid = false, FallbackActive = false.
%   A generated candidate is NOT a plan and is not presented as one.
%
%   Of the 13 inputs only EgoKinematics(1) is consumed. The other 12 inputs and
%   EgoKinematics(2) are structurally present and intentionally unread; no
%   artificial reference is added to make them appear used.

% Stage 2 (Plan_Feasibility) consumes CandV, CandCurv, CandValid.
% CandX/CandY are exposed for Stage 3 envelope evaluation and are unused here.
[CandX, CandY, CandV, CandCurv, CandValid] = gen_candidates(EgoKinematics);

NH = 11;
TrajX              = zeros(NH,1);
TrajY              = zeros(NH,1);
TrajV              = zeros(NH,1);
TrajCurv           = zeros(NH,1);
TrajValid          = false;
ManoeuvreLabel     = uint8(0);
FallbackActive     = false;
NumFeasible        = uint16(0);
NumClear           = uint16(0);
NumTracksEvaluated = uint16(0);
RejectIDs          = zeros(32,1,'uint32');
PlanStale          = false;
end

function [CandX, CandY, CandV, CandCurv, CandValid] = gen_candidates(EgoKinematics) %#codegen
%GEN_CANDIDATES  Stage-1 candidate generator. Fixed size, codegen safe.
%
%   No find / unique / sort / cell / persistent / varsize / dynamic growth.
%   The curvature solver is a FIXED 80-iteration bisection - no root-finding
%   function, no data-dependent loop bound.
%
% LONGITUDINAL MODEL (approved D3) - constant acceleration, no reverse travel
%     a < 0 and t >= v0/|a| :  s = v0^2/(2|a|)   (frozen),   v = 0
%     otherwise             :  s = v0*t + a*t^2/2,           v = v0 + a*t
%
% LATERAL MODEL (approved D4/D5) - constant curvature reaching y_off at t = 5 s
%     arc:  x(s) = sin(k*s)/k ,  y(s) = (1-cos(k*s))/k = 2*sin^2(k*s/2)/k
%     solve  y(S5) = y_off  for k, where S5 = s(5)
%
%   Substituting u = k*S5 gives  g(u) = (1-cos u)/u = |y_off|/S5.
%   g oscillates with a 2/u envelope, so this has MANY roots. But
%   g'(u) = h(u)/u^2 with h(u) = u*sin(u) - 1 + cos(u), h(0) = 0 and
%   h'(u) = u*cos(u) > 0 on (0,pi/2), so h > 0 up to its first zero USTAR.
%   Hence g is STRICTLY INCREASING on (0,USTAR] and is a bijection onto
%   (0,GMAX]. The root there is unique and is the SMALLEST-|k| root, i.e. the
%   least-curved realisation. Bracketing bisection on [0,USTAR] finds it
%   deterministically.
%
%   Reachability (a GENERATION condition, never a feasibility rejection):
%       |y_off| <= GMAX * S5
%
% ENGINEERING ASSUMPTIONS - PROVISIONAL, NOT MEASURED VEHICLE LIMITS
%   The five accelerations below are Stage-1 candidate-generation assumptions
%   only. They are NOT measured vehicle limits, NOT validated capabilities,
%   NOT safety-certified, NOT experimentally established, and they do NOT
%   become the Stage-2 dynamic-feasibility limits, which must be defined and
%   validated independently. They require their own sensitivity analysis.
%   -8.0 is NOT justified by ICE U_ego = 8.0; that parameter is not reused here.
%   'hold' is approximately constant speed; 'coast' is a simplified candidate
%   deceleration assumption, NOT a powertrain or drag model.

MAXC = 35;
NH   = 11;
TH   = [0 0.5 1.0 1.5 2.0 2.5 3.0 3.5 4.0 4.5 5.0];
ACC  = [-8.0 -5.0 -1.0 0.0 2.0];
OFF  = [-3.0 -1.75 -0.9 0.0 0.9 1.75 3.0];

USTAR     = 2.331122370414422;      % first root of u*sin(u) + cos(u) = 1
GMAX      = 0.724611353776709;      % g(USTAR), max lateral offset per unit arc
NBIS      = 80;                     % fixed iteration count
KAPPA_EPS = 1e-12;                  % straight-line guard [1/m]

CandX     = zeros(MAXC,NH);
CandY     = zeros(MAXC,NH);
CandV     = zeros(MAXC,NH);
CandCurv  = zeros(MAXC,NH);
CandValid = false(MAXC,1);

v0 = EgoKinematics(1);
if ~isfinite(v0)
    return
end
if v0 < 0
    v0 = 0;
end
% EgoKinematics(2) is deliberately NOT read (D6). Keeping the nominal straight
% preserves compatibility with ICE decision D4, whose M_adm field is computed
% about a straight nominal, so Stage 3 can compare equivalent geometric points.

for ia = 1:5
    a = ACC(ia);
    for io = 1:7
        c = (ia-1)*7 + io;
        y = OFF(io);

        sArr = zeros(1,NH);
        vArr = zeros(1,NH);
        for n = 1:NH
            t = TH(n);
            if a < 0
                ts = v0/(-a);
                if t >= ts
                    sArr(n) = v0*v0/(2*(-a));
                    vArr(n) = 0;
                else
                    sArr(n) = v0*t + 0.5*a*t*t;
                    vArr(n) = v0 + a*t;
                end
            else
                sArr(n) = v0*t + 0.5*a*t*t;
                vArr(n) = v0 + a*t;
            end
        end
        S5 = sArr(NH);

        kmag = 0;
        sgn  = 0;
        ok   = false;
        if y == 0
            ok = true;
        elseif S5 > 0
            cc = abs(y)/S5;
            if cc <= GMAX
                lo = 0;
                hi = USTAR;
                for ib = 1:NBIS
                    m  = 0.5*(lo+hi);
                    sh = sin(0.5*m);
                    if m > 0
                        gv = 2*sh*sh/m;
                    else
                        gv = 0;
                    end
                    if gv < cc
                        lo = m;
                    else
                        hi = m;
                    end
                end
                kmag = 0.5*(lo+hi)/S5;
                ok   = true;
                if y > 0
                    sgn = 1;
                else
                    sgn = -1;
                end
            end
        end
        CandValid(c) = ok;

        if ok
            for n = 1:NH
                if kmag > KAPPA_EPS
                    ks = kmag*sArr(n);
                    sh = sin(0.5*ks);
                    xx = sin(ks)/kmag;
                    yy = 2*sh*sh/kmag;
                else
                    xx = sArr(n);
                    yy = 0;
                end
                CandX(c,n)    = xx;
                CandY(c,n)    = sgn*yy;
                CandV(c,n)    = vArr(n);
                CandCurv(c,n) = sgn*kmag;
            end
        end
    end
end
end

== matlab function ADAS_Main/LiDAR_Perception/LiDAR_Feature_Extraction/LiDAR_Preprocess ==
  data: loc input; xyzOut output; intensityIn input; isValid input; intensityOut output; validMask output; xyzSensor output
function [xyzOut, intensityOut, validMask, xyzSensor] = LiDAR_Preprocess( ...
    loc, intensityIn, isValid)

xyzSensor = loc;

% LiDAR sensor position relative to ego reference frame
sensorPos = [1.5 0 1.6];
% Ego vehicle exclusion box
xmin = -1.15;
xmax =  3.85;

ymin = -1.05;
ymax =  1.05;

zmin = -0.10;
zmax =  1.55;

% Sensor-frame -> Ego-frame transformation
xyzOut = loc;

xyzOut(:,:,1,:) = loc(:,:,1,:) + sensorPos(1);
xyzOut(:,:,2,:) = loc(:,:,2,:) + sensorPos(2);
xyzOut(:,:,3,:) = loc(:,:,3,:) + sensorPos(3);

% Start with a per-point mask controlled by sensor validity
validMask = false(size(xyzOut,1), size(xyzOut,2));

if isValid
    validMask = isfinite(xyzOut(:,:,1)) & ...
        isfinite(xyzOut(:,:,2)) & ...
        isfinite(xyzOut(:,:,3));
end

% Remove points belonging to the ego vehicle
egoMask = ...
    (xyzOut(:,:,1,:) >= xmin) & (xyzOut(:,:,1,:) <= xmax) & ...
    (xyzOut(:,:,2,:) >= ymin) & (xyzOut(:,:,2,:) <= ymax) & ...
    (xyzOut(:,:,3,:) >= zmin) & (xyzOut(:,:,3,:) <= zmax);

validMask = validMask & ~egoMask;

% Preserve intensity
intensityOut = intensityIn;

end
